simulink model "SingleTrack_RTW"  (Simulink 9.3)
settings: Solver=ode1  StartTime=0.0  StopTime=inf  FixedStep=0.001  RelTol=1e-3
PreLoadFcn:
  | vehicle = 'Car'; if ~length(which('cmcmd')), cmenv; end
  | SingleTrack_RTW_bus
  | SingleTrack_RTW_params
InitFcn:
  | vehicle = 'Car'; if ~length(which('cmcmd')), cmenv; end
  | SingleTrack_RTW_bus
undefined symbols (not defined in the file): Car_Bdy1_mass, Car_Steering_i, Car_Whl_Radius, Car_WhlBaseF, Car_WhlBaseR, mEngineMax, PT_DL_iDiff, PT_GearBox_iForwardGears
libraries: CarMaker4SL x7
(part 3 of 3)

== system SingleTrack_RTW/SingleTrack/CreateBus Vhcl.Fr1/Tr2Fr0/Subsystem_02 ==
  sincos : Inport
  Add : Sum
  Bus Selector : BusSelector  OutputSignals=crx,sry,crz,srx,srz
  Product : Product  Inputs=3  RndMeth=Zero
  Product1 : Product  RndMeth=Zero
  Tr2Fr1_02 : Outport
  wires:
  Bus Selector/4 -> Product1/1  "<srx>"
  Bus Selector/5 -> Product1/2  "<srz>"
  Bus Selector/3 -> Product/3  "<crz>"
  Bus Selector/2 -> Product/2  "<sry>"
  Bus Selector/1 -> Product/1  "<crx>"
  sincos/1 -> Bus Selector/1
  Product/1 -> Add/1
  Product1/1 -> Add/2
  Add/1 -> Tr2Fr1_02/1

== system SingleTrack_RTW/SingleTrack/CreateBus Vhcl.Fr1/Tr2Fr0/Subsystem_10 ==
  sincos : Inport
  Bus Selector : BusSelector  OutputSignals=cry,srz
  Product : Product  RndMeth=Zero
  Tr2Fr1_10 : Outport
  wires:
  sincos/1 -> Bus Selector/1
  Product/1 -> Tr2Fr1_10/1
  Bus Selector/1 -> Product/1  "<cry>"
  Bus Selector/2 -> Product/2  "<srz>"

== system SingleTrack_RTW/SingleTrack/CreateBus Vhcl.Fr1/Tr2Fr0/Subsystem_11 ==
  sincos : Inport
  Add : Sum
  Bus Selector : BusSelector  OutputSignals=srx,sry,srz,crx,crz
  Product : Product  Inputs=3  RndMeth=Zero
  Product1 : Product  RndMeth=Zero
  Tr2Fr1_11 : Outport
  wires:
  Bus Selector/4 -> Product1/1  "<crx>"
  Bus Selector/5 -> Product1/2  "<crz>"
  Bus Selector/3 -> Product/3  "<srz>"
  Bus Selector/2 -> Product/2  "<sry>"
  Bus Selector/1 -> Product/1  "<srx>"
  Add/1 -> Tr2Fr1_11/1
  Product1/1 -> Add/2
  Product/1 -> Add/1
  sincos/1 -> Bus Selector/1

== system SingleTrack_RTW/SingleTrack/CreateBus Vhcl.Fr1/Tr2Fr0/Subsystem_12 ==
  sincos : Inport
  Add : Sum  Inputs=+-
  Bus Selector : BusSelector  OutputSignals=crx,sry,srz,srx,crz
  Product : Product  Inputs=3  RndMeth=Zero
  Product1 : Product  RndMeth=Zero
  Tr2Fr1_12 : Outport
  wires:
  Bus Selector/4 -> Product1/1  "<srx>"
  Bus Selector/5 -> Product1/2  "<crz>"
  Bus Selector/3 -> Product/3  "<srz>"
  Bus Selector/2 -> Product/2  "<sry>"
  Bus Selector/1 -> Product/1  "<crx>"
  sincos/1 -> Bus Selector/1
  Product/1 -> Add/1
  Product1/1 -> Add/2
  Add/1 -> Tr2Fr1_12/1

== system SingleTrack_RTW/SingleTrack/CreateBus Vhcl.Fr1/Tr2Fr0/Subsystem_20 ==
  sincos : Inport
  Bus Selector : BusSelector  OutputSignals=sry
  Gain : Gain  Gain=-1
  Tr2Fr1_20 : Outport
  wires:
  Bus Selector/1 -> Gain/1  "<sry>"
  Gain/1 -> Tr2Fr1_20/1
  sincos/1 -> Bus Selector/1

== system SingleTrack_RTW/SingleTrack/CreateBus Vhcl.Fr1/Tr2Fr0/Subsystem_21 ==
  sincos : Inport
  Bus Selector : BusSelector  OutputSignals=srx,cry
  Product : Product  RndMeth=Zero
  Tr2Fr1_21 : Outport
  wires:
  Bus Selector/2 -> Product/2  "<cry>"
  Bus Selector/1 -> Product/1  "<srx>"
  Product/1 -> Tr2Fr1_21/1
  sincos/1 -> Bus Selector/1

== system SingleTrack_RTW/SingleTrack/CreateBus Vhcl.Fr1/Tr2Fr0/Subsystem_22 ==
  sincos : Inport
  Bus Selector : BusSelector  OutputSignals=crx,cry
  Product : Product  RndMeth=Zero
  Tr2Fr1_22 : Outport
  wires:
  Bus Selector/2 -> Product/2  "<cry>"
  Bus Selector/1 -> Product/1  "<crx>"
  sincos/1 -> Bus Selector/1
  Product/1 -> Tr2Fr1_22/1

== system SingleTrack_RTW/SingleTrack/CreateBus Vhcl.Fr1/Tr2Fr0/sincos ==
  Car : Inport
  Bus Creator : BusCreator  Inputs=6
  Bus Selector : BusSelector  OutputSignals=Road_Fr1_rx,Road_Fr1_ry,Car_Yaw
  Trigonometric Function : Trigonometry
  Trigonometric Function1 : Trigonometry  Operator=cos
  Trigonometric Function2 : Trigonometry
  Trigonometric Function3 : Trigonometry
  Trigonometric Function4 : Trigonometry  Operator=cos
  Trigonometric Function5 : Trigonometry  Operator=cos
  sincos : Outport
  wires:
  Bus Creator/1 -> sincos/1
  Trigonometric Function/1 -> Bus Creator/1  "srx"
  Trigonometric Function3/1 -> Bus Creator/2  "sry"
  Trigonometric Function2/1 -> Bus Creator/3  "srz"
  Trigonometric Function1/1 -> Bus Creator/4  "crx"
  Trigonometric Function4/1 -> Bus Creator/5  "cry"
  Trigonometric Function5/1 -> Bus Creator/6  "crz"
  Car/1 -> Bus Selector/1
  Bus Selector/3 -> Trigonometric Function5/1, Trigonometric Function2/1  "<Car_Yaw>"
  Bus Selector/2 -> Trigonometric Function4/1, Trigonometric Function3/1  "<Road_Fr1_ry>"
  Bus Selector/1 -> Trigonometric Function1/1, Trigonometric Function/1  "<Road_Fr1_rx>"

== system SingleTrack_RTW/SingleTrack/single-track mass point model/Car.v_1/PassIfSim ==
  note: Output original value only when simulating,
      | and zero during pre- or postprocessing.
  In1 : Inport
  "   " : Product  SaturateOnIntegerOverflow=on  InputSameDT=on  OutDataTypeStr=Inherit: Same as first input
  Data Type Conversion : DataTypeConversion
  Out1 : Outport
  wires:
  In1/1 -> "   "/1
  Data Type Conversion/1 -> "   "/2
  "   "/1 -> Out1/1
  [TRSim] -> Data Type Conversion/1

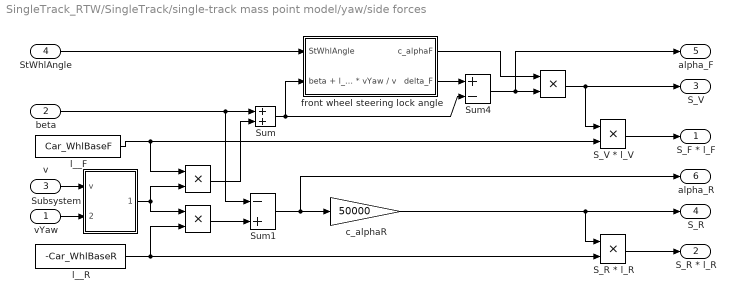
== system SingleTrack_RTW/SingleTrack/single-track mass point model/yaw/side forces ==
  vYaw : Inport
  beta : Inport  Port=2
  v : Inport  Port=3
  StWhlAngle : Inport  Port=4
  " " : Product  SaturateOnIntegerOverflow=on  InputSameDT=on  OutDataTypeStr=Inherit: Same as first input
  "  " : Product  SaturateOnIntegerOverflow=on  InputSameDT=on  OutDataTypeStr=Inherit: Same as first input
  "            " : Product  SaturateOnIntegerOverflow=on  InputSameDT=on  OutDataTypeStr=Inherit: Same as first input
  "S_R * l_R " : Product  SaturateOnIntegerOverflow=on  InputSameDT=on  OutDataTypeStr=Inherit: Same as first input
  "S_V * l_V " : Product  SaturateOnIntegerOverflow=on  InputSameDT=on  OutDataTypeStr=Inherit: Same as first input
  Subsystem : Subsystem
  Sum : Sum  SaturateOnIntegerOverflow=on  InputSameDT=on  OutDataTypeStr=Inherit: Same as first input
  Sum1 : Sum  Inputs=-+  SaturateOnIntegerOverflow=on  InputSameDT=on  OutDataTypeStr=Inherit: Same as first input
  Sum4 : Sum  Inputs=+-  SaturateOnIntegerOverflow=on  InputSameDT=on  OutDataTypeStr=Inherit: Same as first input
  c_alphaR : Gain  Gain=50000  SaturateOnIntegerOverflow=on  OutDataTypeStr=Inherit: Same as input  ParamDataTypeStr=Inherit: Same as input
  front wheel steering lock angle : Subsystem
  l__F : Constant  Value=Car_WhlBaseF
  l__R : Constant  Value=-Car_WhlBaseR
  S_F * l_F : Outport
  S_R * l_R : Outport  Port=2
  S_V : Outport  Port=3
  S_R : Outport  Port=4
  alpha_F : Outport  Port=5
  alpha_R : Outport  Port=6
  wires:
  front wheel steering lock angle/1(c_alphaF) -> "            "/1
  StWhlAngle/1 -> front wheel steering lock angle/1(StWhlAngle)
  "S_R * l_R "/1 -> S_R * l_R/1
  Sum4/1 -> alpha_F/1, "            "/2
  front wheel steering lock angle/2(delta_F) -> Sum4/1
  Sum/1 -> front wheel steering lock angle/2(beta + l_F * vYaw / v), Sum4/2
  v/1 -> Subsystem/1(v)
  vYaw/1 -> Subsystem/2(vYaw)
  "S_V * l_V "/1 -> S_F * l_F/1
  "            "/1 -> S_V/1, "S_V * l_V "/1
  c_alphaR/1 -> S_R/1, "S_R * l_R "/1
  Sum1/1 -> alpha_R/1, c_alphaR/1
  "  "/1 -> Sum/2
  " "/1 -> Sum1/2
  l__R/1 -> "S_R * l_R "/2, " "/2
  Subsystem/1(vYaw/v) -> "  "/2, " "/1
  l__F/1 -> "S_V * l_V "/2, "  "/1
  beta/1 -> Sum/1, Sum1/1

== system SingleTrack_RTW/SingleTrack/single-track mass point model/yaw/sideslip angle ==
  vYaw : Inport
  m : Inport  Port=2
  v_dot : Inport  Port=3
  v : Inport  Port=4
  S : Inport  Port=5
  " " : Product  Inputs=*/  SaturateOnIntegerOverflow=on  InputSameDT=on  OutDataTypeStr=Inherit: Same as first input
  "  " : Product  SaturateOnIntegerOverflow=on  InputSameDT=on  OutDataTypeStr=Inherit: Same as first input
  Subsystem : Subsystem
  Sum2 : Sum  Inputs=+-  SaturateOnIntegerOverflow=on  InputSameDT=on  OutDataTypeStr=Inherit: Same as first input
  beta_dot * dt : Integrator  ExternalReset=level
  beta_dot : Outport
  beta : Outport  Port=2
  wires:
  v/1 -> Subsystem/2(v)
  Subsystem/1(Out1) -> beta_dot/1, beta_dot * dt/1
  vYaw/1 -> Subsystem/1(vYaw)
  Sum2/1 -> Subsystem/3(In3)
  "  "/1 -> Sum2/2
  m/1 -> " "/2
  v_dot/1 -> "  "/1
  " "/1 -> Sum2/1
  S/1 -> " "/1
  beta_dot * dt/1 -> "  "/2, beta/1
  [TRStart] -> beta_dot * dt/2

== system SingleTrack_RTW/SingleTrack/single-track mass point model/yaw/side forces/Subsystem ==
  v : Inport
  vYaw : Inport  Port=2
  If : If  IfExpression=u1 > 0.1 | u1 < -0.1
  If Action Subsystem : Subsystem  TreatAsAtomicUnit=on
  If Action Subsystem1 : Subsystem  TreatAsAtomicUnit=on
  Merge : Merge  InitialOutput=0
  vYaw/v : Outport
  wires:
  v/1 -> If Action Subsystem/1(v), If/1
  vYaw/1 -> If Action Subsystem/2(vYaw)
  If/1 -> If Action Subsystem/Action
  If/2 -> If Action Subsystem1/Action
  Merge/1 -> vYaw/v/1
  If Action Subsystem/1(Out1) -> Merge/1
  If Action Subsystem1/1(Out1) -> Merge/2

== system SingleTrack_RTW/SingleTrack/single-track mass point model/yaw/side forces/front wheel steering lock angle ==
  StWhlAngle : Inport
  beta + l_F * vYaw / v : Inport  Port=2
  "   " : Product  SaturateOnIntegerOverflow=on  InputSameDT=on  OutDataTypeStr=Inherit: Same as first input
  "     " : Constant
  "      " : Product  Inputs=*/  SaturateOnIntegerOverflow=on  InputSameDT=on  OutDataTypeStr=Inherit: Same as first input
  "       " : Product  Inputs=*/*  SaturateOnIntegerOverflow=on  InputSameDT=on  OutDataTypeStr=Inherit: Same as first input
  1/ i_S : Gain  Gain=1/Car_Steering_i  SaturateOnIntegerOverflow=on  OutDataTypeStr=Inherit: Same as input  ParamDataTypeStr=Inherit: Same as input
  C_S : Constant  Value=10000
  Sum2 : Sum  SaturateOnIntegerOverflow=on  InputSameDT=on  OutDataTypeStr=Inherit: Same as first input
  Sum3 : Sum  SaturateOnIntegerOverflow=on  InputSameDT=on  OutDataTypeStr=Inherit: Same as first input
  "c_alphaF " : Constant  Value=50000
  n_F : Constant  Value=0.06
  c_alphaF : Outport
  delta_F : Outport  Port=2
  wires:
  "      "/1 -> delta_F/1
  "c_alphaF "/1 -> "       "/1, c_alphaF/1
  n_F/1 -> "       "/3
  C_S/1 -> "       "/2
  Sum2/1 -> "      "/1
  Sum3/1 -> "      "/2
  "     "/1 -> Sum3/1
  1/ i_S/1 -> Sum2/1
  "   "/1 -> Sum2/2
  StWhlAngle/1 -> 1/ i_S/1
  "       "/1 -> "   "/1, Sum3/2
  beta + l_F * vYaw / v/1 -> "   "/2

== system SingleTrack_RTW/SingleTrack/single-track mass point model/yaw/sideslip angle/Subsystem ==
  vYaw : Inport
  v : Inport  Port=2
  In3 : Inport  Port=3
  If : If  IfExpression=u1 > 0.1 | u1 < -0.1
  If Action Subsystem : Subsystem  TreatAsAtomicUnit=on
  If Action Subsystem1 : Subsystem  TreatAsAtomicUnit=on
  Merge : Merge
  Sum1 : Sum  Inputs=-+  SaturateOnIntegerOverflow=on  InputSameDT=on  OutDataTypeStr=Inherit: Same as first input
  Out1 : Outport
  wires:
  vYaw/1 -> Sum1/1
  v/1 -> If Action Subsystem/1(v), If/1
  Sum1/1 -> Out1/1
  If Action Subsystem/1(Out1) -> Merge/1
  If Action Subsystem1/1(Out1) -> Merge/2
  Merge/1 -> Sum1/2
  If/2 -> If Action Subsystem1/Action
  In3/1 -> If Action Subsystem/2(In3)
  If/1 -> If Action Subsystem/Action

== system SingleTrack_RTW/SingleTrack/single-track mass point model/yaw/side forces/Subsystem/If Action Subsystem ==
  v : Inport
  vYaw : Inport  Port=2
  Action Port : ActionPort  ActionPortLabel=if { }
  vYaw / v : Product  Inputs=/*  SaturateOnIntegerOverflow=on  InputSameDT=on  OutDataTypeStr=Inherit: Same as first input
  Out1 : Outport  InitialOutput=0
  wires:
  v/1 -> vYaw / v/1
  vYaw/1 -> vYaw / v/2
  vYaw / v/1 -> Out1/1

== system SingleTrack_RTW/SingleTrack/single-track mass point model/yaw/side forces/Subsystem/If Action Subsystem1 ==
  Action Port : ActionPort  ActionPortLabel=else { }
  Constant : Constant  Value=0
  Out1 : Outport  InitialOutput=0
  wires:
  Constant/1 -> Out1/1

== system SingleTrack_RTW/SingleTrack/single-track mass point model/yaw/sideslip angle/Subsystem/If Action Subsystem ==
  v : Inport
  In3 : Inport  Port=2
  Action Port : ActionPort  ActionPortLabel=if { }
  "    " : Product  Inputs=/*  SaturateOnIntegerOverflow=on  InputSameDT=on  OutDataTypeStr=Inherit: Same as first input
  Out1 : Outport  InitialOutput=0
  wires:
  v/1 -> "    "/1
  In3/1 -> "    "/2
  "    "/1 -> Out1/1

== system SingleTrack_RTW/SingleTrack/single-track mass point model/yaw/sideslip angle/Subsystem/If Action Subsystem1 ==
  Action Port : ActionPort  ActionPortLabel=else { }
  Constant : Constant  Value=0
  Out1 : Outport  InitialOutput=0
  wires:
  Constant/1 -> Out1/1
